simulink model "trial_v2"  (R2019b)
settings: Solver=VariableStepAuto  StartTime=0.0  StopTime=10.0  RelTol=1e-3
undefined symbols (not defined in the file or in its folder): dd_theta_ref
libraries: simulink x1
settings Model: Creator=arund  LastModifiedBy=arund

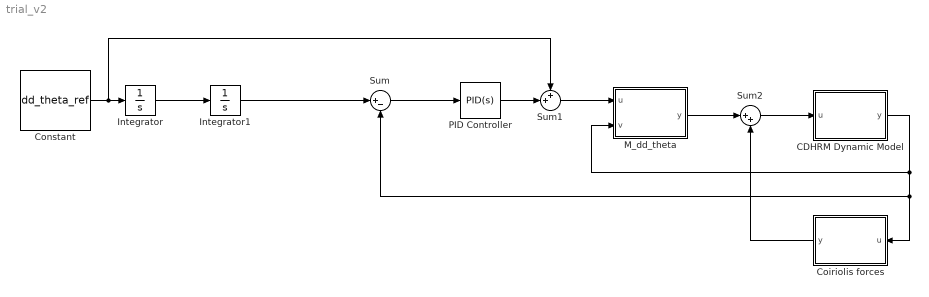
== system trial_v2 ==
  CDHRM Dynamic Model : MATLAB Function  TreatAsAtomicUnit=on
  Coiriolis forces : MATLAB Function  TreatAsAtomicUnit=on
  Constant : Constant  Value=dd_theta_ref
  Integrator : Integrator
  Integrator1 : Integrator
  M_dd_theta : MATLAB Function  TreatAsAtomicUnit=on
  PID Controller : simulink/Continuous/PID Controller  Controller=PID  Form=Parallel  TimeDomain=Continuous-time  SampleTime=-1  IntegratorMethod=Forward Euler  FilterMethod=Forward Euler  ControllerParametersSource=internal  P=1  I=1  D=0  UseFilter=on  N=100  TunerSelectOption=Transfer Function Based (PID Tuner App)  InitialConditionSource=internal  InitialConditionForIntegrator=0  InitialConditionForFilter=0  DifferentiatorICPrevScaledInput=0  ExternalReset=none  TrackingMode=off  Kt=1  LimitOutput=off  UpperSaturationLimit=inf  LowerSaturationLimit=-inf  LinearizeAsGain=on  AntiWindupMode=none  Kb=1  POutMin=[]  POutMax=[]  IOutMin=[]  IOutMax=[]  DOutMin=[]  DOutMax=[]  NOutMin=[]  NOutMax=[]  SumOutMin=[]  SumOutMax=[]  SaturationOutMin=[]  SaturationOutMax=[]  PParamMin=[]  PParamMax=[]  IParamMin=[]  IParamMax=[]  DParamMin=[]  DParamMax=[]  NParamMin=[]  NParamMax=[]  KbParamMin=[]  KbParamMax=[]  KtParamMin=[]  KtParamMax=[]  KbOutMin=[]  KbOutMax=[]  KtOutMin=[]  KtOutMax=[]  IntegratorOutMin=[]  IntegratorOutMax=[]  FilterOutMin=[]  FilterOutMax=[]  SumI1OutMin=[]  SumI1OutMax=[]  SumI2OutMin=[]  SumI2OutMax=[]  SumI3OutMin=[]  SumI3OutMax=[]  SumI4OutMin=[]  SumI4OutMax=[]  SumDOutMin=[]  SumDOutMax=[]  DifferentiatorOutMin=[]  DifferentiatorOutMax=[]  FilterDiffOutCoefMin=[]  FilterDiffOutCoefMax=[]  ReciprocalOutMin=[]  ReciprocalOutMax=[]  SumDenOutMin=[]  SumDenOutMax=[]  SumNumOutMin=[]  SumNumOutMax=[]  DivideOutMin=[]  DivideOutMax=[]  IntegratorContinuousStateAttributes=''  IntegratorStateMustResolveToSignalObject=off  IntegratorRTWStateStorageClass=Auto  FilterContinuousStateAttributes=''  FilterStateMustResolveToSignalObject=off  FilterRTWStateStorageClass=Auto  ParallelPVariant=InternalParameters  IdealPVariant=Disabled  IVariant=InternalParameters  DVariant=InternalParameters  IntegratorVariant=Continuous  SatVariant=Disabled  AWVariant=Passthrough  PCopyVariant=Disabled  TRVariant=Disabled  FdbkBlocksVariant=Forward  IdealPFdbkVariant=Disabled  SatFdbkVariant=Disabled  DerivativeFilterVariant=ContFilter  NVariant=InternalParameters  NCopyVariant=Disabled  FilterICVariant=InternalICsFilter  IntegratorICVariant=InternalICs  ExternalResetVariant=Disabled  TRSumVariant=Passthrough  SumFdbkVariant=Disabled  SumVariant=Sum_PID
  Sum : Sum  Inputs=|+-
  Sum1 : Sum  Inputs=++|
  Sum2 : Sum  Inputs=|++
  wires:
  Sum/1 -> PID Controller/1
  Constant/1 -> Sum1/1, Integrator/1
  Integrator/1 -> Integrator1/1
  Integrator1/1 -> Sum/1
  PID Controller/1 -> Sum1/2
  M_dd_theta/1(y) -> Sum2/1
  Coiriolis forces/1(y) -> Sum2/2
  Sum2/1 -> CDHRM Dynamic Model/1(u)
  CDHRM Dynamic Model/1(y) -> M_dd_theta/2(v), Sum/2, Coiriolis forces/1(u)
  Sum1/1 -> M_dd_theta/1(u)

== matlab function trial_v2/CDHRM Dynamic Model ==
  data: u input; y output
function y = fcn(u)
f_dash = F - R*f_dash
n_dash= P*RF + R*n_dash-R*n + n+T_dash
F=f_dash-R*f_dash
T=n_dash - R*n_dash - (P+P)*f_dash+P*(R*f_dash)
y = u;

== matlab function trial_v2/M_dd_theta ==
  data: u input; y output; v input
function y = fcn(u,v)

y = u;

== matlab function trial_v2/Coiriolis forces ==
  data: u input; y output
function y = fcn(u)

y = u;
